simulink model "openloop_on_ramp_mdl"  (Simulink 4.00)
settings: Solver=ode45  StartTime=0.0  StopTime=1097  RelTol=1e-3
values from neighbouring files (symbols this model uses):
  dt = 1    [openloop_on_ramp.m]    (also in same_ord_1_stand_system_new_old_wor.m)
  stm_alpha = 0.0167    [openloop_on_ramp.m]
  stm_ftd = [7 100 120 60   1100 ... (first row only)    [openloop_on_ramp.m]
  stm_ks = 0.031    [openloop_on_ramp.m]
  stm_ks2 = 0.010    (= 0.01)    [openloop_on_ramp.m]
  stm_ks3 = 0.033    [openloop_on_ramp.m]
  stm_ks4 = 0.024    [openloop_on_ramp.m]
  stm_ks5 = 0.025    [openloop_on_ramp.m]
  z0 = 0    [openloop_on_ramp.m]
settings Model: LastModifiedBy=kontorou

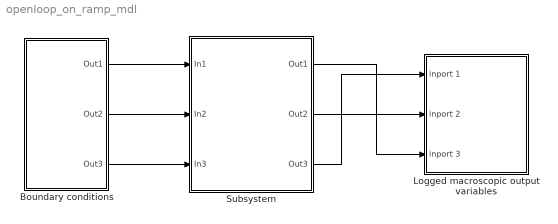
== system openloop_on_ramp_mdl ==
  Boundary conditions : Subsystem
      settings: RTWFcnNameOpts=Auto  RTWFileNameOpts=Auto
      mask Display: disp('Disturbances')
  Logged macroscopic output variables : Subsystem
      settings: RTWFcnNameOpts=Auto  RTWFileNameOpts=Auto
      mask Display: disp('Data')
  Subsystem : Subsystem
      settings: RTWFcnNameOpts=Auto  RTWFileNameOpts=Auto
  wires:
  Subsystem/1(Out1) -> Logged macroscopic output variables/3(inport 3)
  Boundary conditions/1(Out1) -> Subsystem/1(In1)
  Boundary conditions/2(Out2) -> Subsystem/2(In2)
  Subsystem/3(Out3) -> Logged macroscopic output variables/1(inport 1)
  Subsystem/2(Out2) -> Logged macroscopic output variables/2(inport 2)
  Boundary conditions/3(Out3) -> Subsystem/3(In3)

== system openloop_on_ramp_mdl/Boundary conditions ==
  downstream velocity : FromWorkspace  VariableName=[t_in, v_in]  SampleTime=0  OutputAfterFinalValue=Extrapolation
  downstream velocity (km/hour) : ToWorkspace  VariableName=v_in_dt  SampleTime=dt  SaveFormat=Array
  upstream flow : FromWorkspace  VariableName=[t_in, q_in]  SampleTime=0  OutputAfterFinalValue=Extrapolation
  upstream flow1 : FromWorkspace  VariableName=[t_in, q_ramp]  SampleTime=0  OutputAfterFinalValue=Extrapolation
  Out1 : Outport  Port=1
  Out2 : Outport  Port=2
  Out3 : Outport  Port=3
  wires:
  downstream velocity/1 -> Out1/1, downstream velocity (km/hour)/1
  upstream flow/1 -> Out2/1
  upstream flow1/1 -> Out3/1

== system openloop_on_ramp_mdl/Logged macroscopic output variables ==
  inport 1 : Inport  Port=1  LatchInput=off
  inport 2 : Inport  Port=2  LatchInput=off
  inport 3 : Inport  Port=3  LatchInput=off
  Clock : Clock
      settings: DisplayTime=off
  density : ToWorkspace  VariableName=dd  SampleTime=dt  SaveFormat=Array
  flow : ToWorkspace  VariableName=qq  SampleTime=dt  SaveFormat=Array
  time (sample) : ToWorkspace  VariableName=tt  SampleTime=dt  SaveFormat=Array
  velocity : ToWorkspace  VariableName=vv  SampleTime=dt  SaveFormat=Array
  wires:
  inport 3/1 -> velocity/1
  inport 1/1 -> density/1
  inport 2/1 -> flow/1
  Clock/1 -> time (sample)/1

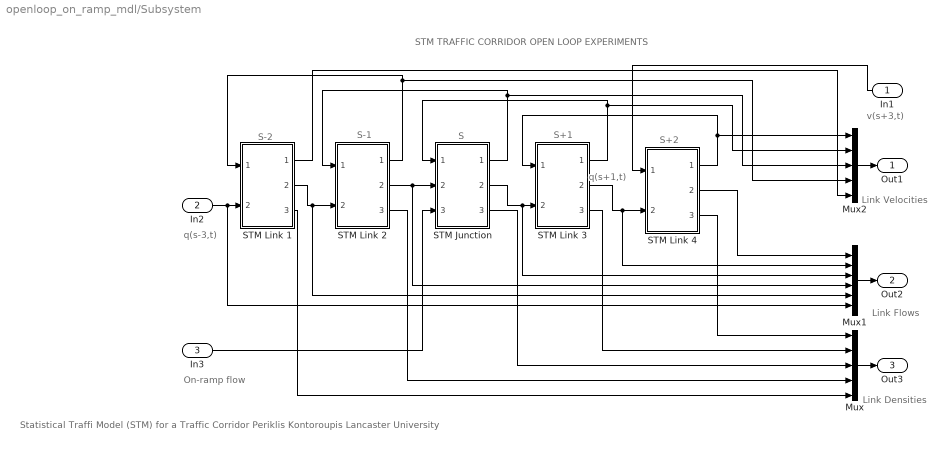
== system openloop_on_ramp_mdl/Subsystem ==
  note: Link
      | Velocities
  note: Link
      | Flows
  note: q(s+1,t)
  note: v(s+3,t)
  note: STM TRAFFIC CORRIDOR OPEN LOOP EXPERIMENTS
  note: On-ramp flow
  note: Link
      | Densities
  note: S-2
  note: S-1
  note: S
  note: S+1
  note: S+2
  note: q(s-3,t)
  note: Statistical Traffi Model (STM)
      | for a Traffic Corridor
      | Periklis Kontoroupis
      | Lancaster University
  In1 : Inport  Orientation=left  Port=1  LatchInput=off
  In2 : Inport  Port=2  LatchInput=off
  In3 : Inport  Port=3  LatchInput=off
  Mux : Mux  Inputs=5
  Mux1 : Mux  Inputs=6
  Mux2 : Mux  Inputs=5
  STM Junction : Subsystem
      settings: RTWFcnNameOpts=Auto  RTWFileNameOpts=Auto
  STM Link 1 : Subsystem
      settings: RTWFcnNameOpts=Auto  RTWFileNameOpts=Auto
  STM Link 2 : Subsystem
      settings: RTWFcnNameOpts=Auto  RTWFileNameOpts=Auto
  STM Link 3 : Subsystem
      settings: RTWFcnNameOpts=Auto  RTWFileNameOpts=Auto
  STM Link 4 : Subsystem
      settings: RTWFcnNameOpts=Auto  RTWFileNameOpts=Auto
  Out1 : Outport  Port=1
  Out2 : Outport  Port=2
  Out3 : Outport  Port=3
  wires:
  STM Link 3/2(link flow (veh/min)) -> STM Link 4/2(upstream flow (veh/min)), Mux1/2
  STM Link 4/1(link velocity (km/hour)) -> STM Link 3/1(downstream velocity (km/hour)), Mux2/1
  Mux1/1 -> Out2/1
  Mux/1 -> Out3/1
  Mux2/1 -> Out1/1
  In2/1 -> STM Link 1/2(upstream flow (veh/min)), Mux1/6
  STM Link 4/2(link flow (veh/min)) -> Mux1/1
  STM Link 4/3(link density (veh/km)) -> Mux/1
  STM Link 3/3(link density (veh/km)) -> Mux/2
  STM Link 1/3(link density (veh/km)) -> Mux/5
  In3/1 -> STM Junction/3(on-ramp flow (veh/min))
  STM Junction/1(link velocity (km/hour)) -> STM Link 2/1(downstream velocity (km/hour)), Mux2/3
  STM Link 2/1(link velocity (km/hour)) -> STM Link 1/1(downstream velocity (km/hour)), Mux2/4
  STM Link 1/2(link flow (veh/min)) -> STM Link 2/2(upstream flow (veh/min)), Mux1/5
  STM Link 2/2(link flow (veh/min)) -> STM Junction/2(upstream flow (veh/min)), Mux1/4
  STM Junction/2(link flow (veh/min)) -> STM Link 3/2(upstream flow (veh/min)), Mux1/3
  STM Link 3/1(link velocity (km/hour)) -> STM Junction/1(downstream velocity (km/hour)), Mux2/2
  STM Link 2/3(link density (veh/km)) -> Mux/4
  STM Junction/3(link density (veh/km)) -> Mux/3
  In1/1 -> STM Link 4/1(downstream velocity (km/hour))
  STM Link 1/1(link velocity (km/hour)) -> Mux2/5

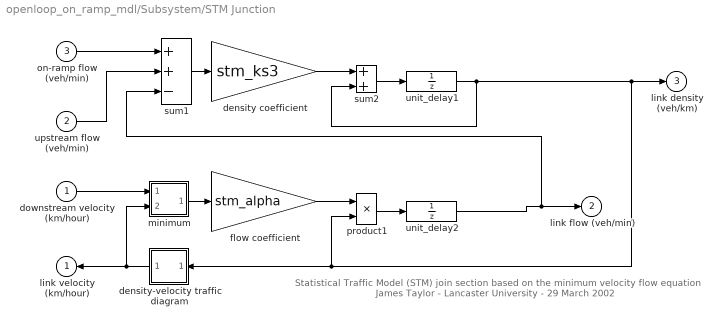
== system openloop_on_ramp_mdl/Subsystem/STM Junction ==
  note: Statistical Traffic Model (STM) join section
      | based on the minimum velocity flow equation
      | James Taylor - Lancaster University - 29 March 2002
  downstream velocity (km/hour) : Inport  Port=1  LatchInput=off
  upstream flow (veh/min) : Inport  Port=2  LatchInput=off
  on-ramp flow (veh/min) : Inport  Port=3  LatchInput=off
  density coefficient : Gain  Gain=stm_ks3  Multiplication=Element-wise(K.*u)  SaturateOnIntegerOverflow=on
  density-velocity traffic diagram : Subsystem  Orientation=left  mask(Fundamental Traffic Diagram){v1=stm_ftd(3,1), v2=stm_ftd(3,2), v3=stm_ftd(3,3), r1=stm_ftd(3,4), r3=stm_ftd(3,5)}
      mask prompts: v1 "Minimum velocity:"; v2 "Critical velocity:"; v3 "Maximum velocity:"; r1 "Critical density:"; r3 "Theoretical density for zero velocity:"
      mask help: Traffic diagram for density-velocity relationship.
      settings: RTWFcnNameOpts=Auto  RTWFileNameOpts=Auto
      mask Help: Connect traffic density to the input and velocity to the output. Based on figure 4 of J. Whittaker, S. Garside and K. Lindveld (1997) Tracking and predicting a network traffic process, International Journal of Forecasting 13, 51-61.
      mask Display: disp('FTD')
  flow coefficient : Gain  Gain=stm_alpha  Multiplication=Element-wise(K.*u)  SaturateOnIntegerOverflow=on
  minimum : Subsystem
      settings: RTWFcnNameOpts=Auto  RTWFileNameOpts=Auto
      mask Type: Minimum
      mask Description: Selects minimum of two inputs.
      mask Help: The output of this block is the minimum of the two input signals.
      mask Display: disp('MIN')
  product1 : Product  Inputs=2  Multiplication=Element-wise(.*)  SaturateOnIntegerOverflow=on
  sum1 : Sum  Inputs=++-  SaturateOnIntegerOverflow=on
  sum2 : Sum  Inputs=++  SaturateOnIntegerOverflow=on
  unit_delay1 : UnitDelay  X0=z0  SampleTime=dt
      settings: RTWStateStorageClass=Auto
  unit_delay2 : UnitDelay  X0=z0  SampleTime=dt
      settings: RTWStateStorageClass=Auto
  link velocity (km/hour) : Outport  Orientation=left  Port=1
  link flow (veh/min) : Outport  Port=2
  link density (veh/km) : Outport  Port=3
  wires:
  on-ramp flow (veh/min)/1 -> sum1/1
  upstream flow (veh/min)/1 -> sum1/2
  flow coefficient/1 -> product1/1
  product1/1 -> unit_delay2/1
  downstream velocity (km/hour)/1 -> minimum/1(inport1)
  unit_delay2/1 -> link flow (veh/min)/1, sum1/3
  sum1/1 -> density coefficient/1
  minimum/1(outport) -> flow coefficient/1
  unit_delay1/1 -> product1/2, density-velocity traffic diagram/1(density), link density (veh/km)/1, sum2/2
  density coefficient/1 -> sum2/1
  sum2/1 -> unit_delay1/1
  density-velocity traffic diagram/1(velocity) -> minimum/2(inport2), link velocity (km/hour)/1

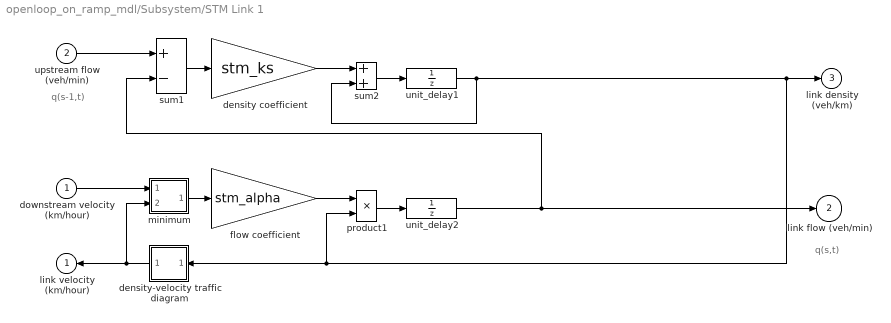
== system openloop_on_ramp_mdl/Subsystem/STM Link 1 ==
  note: q(s-1,t)
  note: q(s,t)
  downstream velocity (km/hour) : Inport  Port=1  LatchInput=off
  upstream flow (veh/min) : Inport  Port=2  LatchInput=off
  density coefficient : Gain  Gain=stm_ks  Multiplication=Element-wise(K.*u)  SaturateOnIntegerOverflow=on
  density-velocity traffic diagram : Subsystem  Orientation=left  mask(Fundamental Traffic Diagram){v1=stm_ftd(1,1), v2=stm_ftd(1,2), v3=stm_ftd(1,3), r1=stm_ftd(1,4), r3=stm_ftd(1,5)}
      mask prompts: v1 "Minimum velocity:"; v2 "Critical velocity:"; v3 "Maximum velocity:"; r1 "Critical density:"; r3 "Theoretical density for zero velocity:"
      mask help: Traffic diagram for density-velocity relationship.
      settings: RTWFcnNameOpts=Auto  RTWFileNameOpts=Auto
      mask Help: Connect traffic density to the input and velocity to the output. Based on figure 4 of J. Whittaker, S. Garside and K. Lindveld (1997) Tracking and predicting a network traffic process, International Journal of Forecasting 13, 51-61.
      mask Display: disp('FTD')
  flow coefficient : Gain  Gain=stm_alpha  Multiplication=Element-wise(K.*u)  SaturateOnIntegerOverflow=on
  minimum : Subsystem
      settings: RTWFcnNameOpts=Auto  RTWFileNameOpts=Auto
      mask Type: Minimum
      mask Description: Selects minimum of two inputs.
      mask Help: The output of this block is the minimum of the two input signals.
      mask Display: disp('MIN')
  product1 : Product  Inputs=2  Multiplication=Element-wise(.*)  SaturateOnIntegerOverflow=on
  sum1 : Sum  Inputs=+-  SaturateOnIntegerOverflow=on
  sum2 : Sum  Inputs=++  SaturateOnIntegerOverflow=on
  unit_delay1 : UnitDelay  X0=z0  SampleTime=dt
      settings: RTWStateStorageClass=Auto
  unit_delay2 : UnitDelay  X0=z0  SampleTime=dt
      settings: RTWStateStorageClass=Auto
  link velocity (km/hour) : Outport  Orientation=left  Port=1
  link flow (veh/min) : Outport  Port=2
  link density (veh/km) : Outport  Port=3
  wires:
  flow coefficient/1 -> product1/1
  product1/1 -> unit_delay2/1
  downstream velocity (km/hour)/1 -> minimum/1(inport1)
  unit_delay2/1 -> sum1/2, link flow (veh/min)/1
  sum1/1 -> density coefficient/1
  minimum/1(outport) -> flow coefficient/1
  unit_delay1/1 -> product1/2, density-velocity traffic diagram/1(density), link density (veh/km)/1, sum2/2
  density coefficient/1 -> sum2/1
  sum2/1 -> unit_delay1/1
  density-velocity traffic diagram/1(velocity) -> minimum/2(inport2), link velocity (km/hour)/1
  upstream flow (veh/min)/1 -> sum1/1

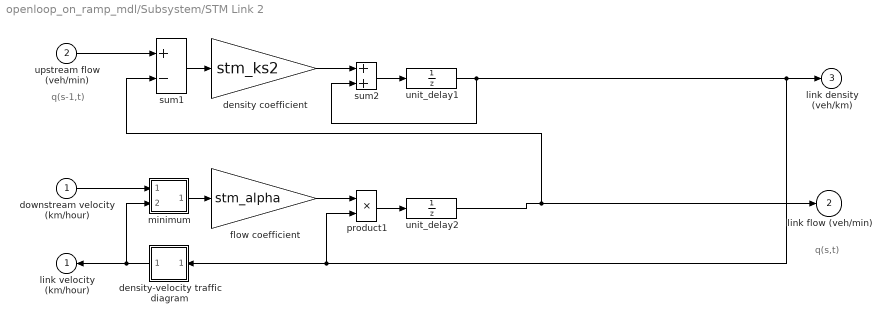
== system openloop_on_ramp_mdl/Subsystem/STM Link 2 ==
  note: q(s-1,t)
  note: q(s,t)
  downstream velocity (km/hour) : Inport  Port=1  LatchInput=off
  upstream flow (veh/min) : Inport  Port=2  LatchInput=off
  density coefficient : Gain  Gain=stm_ks2  Multiplication=Element-wise(K.*u)  SaturateOnIntegerOverflow=on
  density-velocity traffic diagram : Subsystem  Orientation=left  mask(Fundamental Traffic Diagram){v1=stm_ftd(2,1), v2=stm_ftd(2,2), v3=stm_ftd(2,3), r1=stm_ftd(2,4), r3=stm_ftd(2,5)}
      mask prompts: v1 "Minimum velocity:"; v2 "Critical velocity:"; v3 "Maximum velocity:"; r1 "Critical density:"; r3 "Theoretical density for zero velocity:"
      mask help: Traffic diagram for density-velocity relationship.
      settings: RTWFcnNameOpts=Auto  RTWFileNameOpts=Auto
      mask Help: Connect traffic density to the input and velocity to the output. Based on figure 4 of J. Whittaker, S. Garside and K. Lindveld (1997) Tracking and predicting a network traffic process, International Journal of Forecasting 13, 51-61.
      mask Display: disp('FTD')
  flow coefficient : Gain  Gain=stm_alpha  Multiplication=Element-wise(K.*u)  SaturateOnIntegerOverflow=on
  minimum : Subsystem
      settings: RTWFcnNameOpts=Auto  RTWFileNameOpts=Auto
      mask Type: Minimum
      mask Description: Selects minimum of two inputs.
      mask Help: The output of this block is the minimum of the two input signals.
      mask Display: disp('MIN')
  product1 : Product  Inputs=2  Multiplication=Element-wise(.*)  SaturateOnIntegerOverflow=on
  sum1 : Sum  Inputs=+-  SaturateOnIntegerOverflow=on
  sum2 : Sum  Inputs=++  SaturateOnIntegerOverflow=on
  unit_delay1 : UnitDelay  X0=z0  SampleTime=dt
      settings: RTWStateStorageClass=Auto
  unit_delay2 : UnitDelay  X0=z0  SampleTime=dt
      settings: RTWStateStorageClass=Auto
  link velocity (km/hour) : Outport  Orientation=left  Port=1
  link flow (veh/min) : Outport  Port=2
  link density (veh/km) : Outport  Port=3
  wires:
  flow coefficient/1 -> product1/1
  product1/1 -> unit_delay2/1
  downstream velocity (km/hour)/1 -> minimum/1(inport1)
  unit_delay2/1 -> sum1/2, link flow (veh/min)/1
  sum1/1 -> density coefficient/1
  minimum/1(outport) -> flow coefficient/1
  unit_delay1/1 -> product1/2, density-velocity traffic diagram/1(density), link density (veh/km)/1, sum2/2
  density coefficient/1 -> sum2/1
  sum2/1 -> unit_delay1/1
  density-velocity traffic diagram/1(velocity) -> minimum/2(inport2), link velocity (km/hour)/1
  upstream flow (veh/min)/1 -> sum1/1

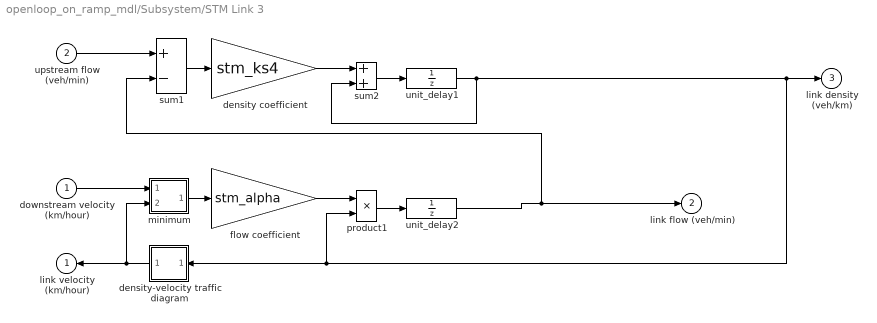
== system openloop_on_ramp_mdl/Subsystem/STM Link 3 ==
  downstream velocity (km/hour) : Inport  Port=1  LatchInput=off
  upstream flow (veh/min) : Inport  Port=2  LatchInput=off
  density coefficient : Gain  Gain=stm_ks4  Multiplication=Element-wise(K.*u)  SaturateOnIntegerOverflow=on
  density-velocity traffic diagram : Subsystem  Orientation=left  mask(Fundamental Traffic Diagram){v1=stm_ftd(4,1), v2=stm_ftd(4,2), v3=stm_ftd(4,3), r1=stm_ftd(4,4), r3=stm_ftd(4,5)}
      mask prompts: v1 "Minimum velocity:"; v2 "Critical velocity:"; v3 "Maximum velocity:"; r1 "Critical density:"; r3 "Theoretical density for zero velocity:"
      mask help: Traffic diagram for density-velocity relationship.
      settings: RTWFcnNameOpts=Auto  RTWFileNameOpts=Auto
      mask Help: Connect traffic density to the input and velocity to the output. Based on figure 4 of J. Whittaker, S. Garside and K. Lindveld (1997) Tracking and predicting a network traffic process, International Journal of Forecasting 13, 51-61.
      mask Display: disp('FTD')
  flow coefficient : Gain  Gain=stm_alpha  Multiplication=Element-wise(K.*u)  SaturateOnIntegerOverflow=on
  minimum : Subsystem
      settings: RTWFcnNameOpts=Auto  RTWFileNameOpts=Auto
      mask Type: Minimum
      mask Description: Selects minimum of two inputs.
      mask Help: The output of this block is the minimum of the two input signals.
      mask Display: disp('MIN')
  product1 : Product  Inputs=2  Multiplication=Element-wise(.*)  SaturateOnIntegerOverflow=on
  sum1 : Sum  Inputs=+-  SaturateOnIntegerOverflow=on
  sum2 : Sum  Inputs=++  SaturateOnIntegerOverflow=on
  unit_delay1 : UnitDelay  X0=z0  SampleTime=dt
      settings: RTWStateStorageClass=Auto
  unit_delay2 : UnitDelay  X0=z0  SampleTime=dt
      settings: RTWStateStorageClass=Auto
  link velocity (km/hour) : Outport  Orientation=left  Port=1
  link flow (veh/min) : Outport  Port=2
  link density (veh/km) : Outport  Port=3
  wires:
  flow coefficient/1 -> product1/1
  product1/1 -> unit_delay2/1
  downstream velocity (km/hour)/1 -> minimum/1(inport1)
  sum1/1 -> density coefficient/1
  minimum/1(outport) -> flow coefficient/1
  unit_delay1/1 -> product1/2, density-velocity traffic diagram/1(density), link density (veh/km)/1, sum2/2
  density coefficient/1 -> sum2/1
  sum2/1 -> unit_delay1/1
  density-velocity traffic diagram/1(velocity) -> minimum/2(inport2), link velocity (km/hour)/1
  unit_delay2/1 -> sum1/2, link flow (veh/min)/1
  upstream flow (veh/min)/1 -> sum1/1

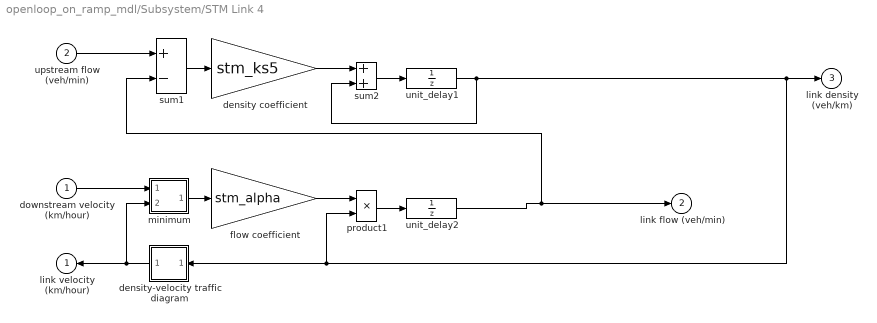
== system openloop_on_ramp_mdl/Subsystem/STM Link 4 ==
  downstream velocity (km/hour) : Inport  Port=1  LatchInput=off
  upstream flow (veh/min) : Inport  Port=2  LatchInput=off
  density coefficient : Gain  Gain=stm_ks5  Multiplication=Element-wise(K.*u)  SaturateOnIntegerOverflow=on
  density-velocity traffic diagram : Subsystem  Orientation=left  mask(Fundamental Traffic Diagram){v1=stm_ftd(5,1), v2=stm_ftd(5,2), v3=stm_ftd(5,3), r1=stm_ftd(5,4), r3=stm_ftd(5,5)}
      mask prompts: v1 "Minimum velocity:"; v2 "Critical velocity:"; v3 "Maximum velocity:"; r1 "Critical density:"; r3 "Theoretical density for zero velocity:"
      mask help: Traffic diagram for density-velocity relationship.
      settings: RTWFcnNameOpts=Auto  RTWFileNameOpts=Auto
      mask Help: Connect traffic density to the input and velocity to the output. Based on figure 4 of J. Whittaker, S. Garside and K. Lindveld (1997) Tracking and predicting a network traffic process, International Journal of Forecasting 13, 51-61.
      mask Display: disp('FTD')
  flow coefficient : Gain  Gain=stm_alpha  Multiplication=Element-wise(K.*u)  SaturateOnIntegerOverflow=on
  minimum : Subsystem
      settings: RTWFcnNameOpts=Auto  RTWFileNameOpts=Auto
      mask Type: Minimum
      mask Description: Selects minimum of two inputs.
      mask Help: The output of this block is the minimum of the two input signals.
      mask Display: disp('MIN')
  product1 : Product  Inputs=2  Multiplication=Element-wise(.*)  SaturateOnIntegerOverflow=on
  sum1 : Sum  Inputs=+-  SaturateOnIntegerOverflow=on
  sum2 : Sum  Inputs=++  SaturateOnIntegerOverflow=on
  unit_delay1 : UnitDelay  X0=z0  SampleTime=dt
      settings: RTWStateStorageClass=Auto
  unit_delay2 : UnitDelay  X0=z0  SampleTime=dt
      settings: RTWStateStorageClass=Auto
  link velocity (km/hour) : Outport  Orientation=left  Port=1
  link flow (veh/min) : Outport  Port=2
  link density (veh/km) : Outport  Port=3
  wires:
  flow coefficient/1 -> product1/1
  product1/1 -> unit_delay2/1
  downstream velocity (km/hour)/1 -> minimum/1(inport1)
  unit_delay2/1 -> sum1/2, link flow (veh/min)/1
  sum1/1 -> density coefficient/1
  minimum/1(outport) -> flow coefficient/1
  unit_delay1/1 -> product1/2, density-velocity traffic diagram/1(density), link density (veh/km)/1, sum2/2
  density coefficient/1 -> sum2/1
  sum2/1 -> unit_delay1/1
  density-velocity traffic diagram/1(velocity) -> minimum/2(inport2), link velocity (km/hour)/1
  upstream flow (veh/min)/1 -> sum1/1

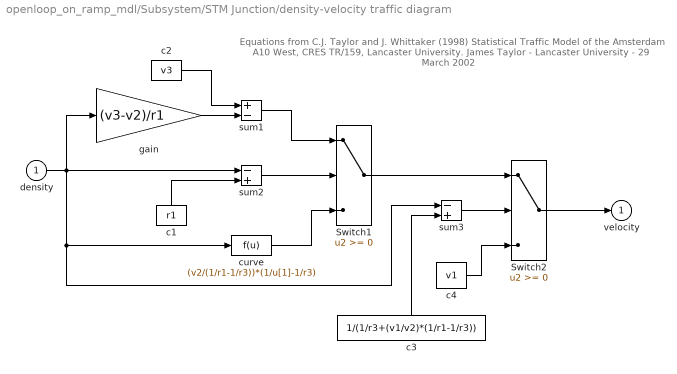
== system openloop_on_ramp_mdl/Subsystem/STM Junction/density-velocity traffic diagram ==
  note: Equations from C.J. Taylor and J. Whittaker (1998) Statistical Traffic Model
      | of the Amsterdam A10 West, CRES TR/159, Lancaster University.
      | James Taylor - Lancaster University - 29 March 2002
  density : Inport  Port=1  LatchInput=off
  Switch1 : Switch  Threshold=0
  Switch2 : Switch  Threshold=0
  c1 : Constant  Orientation=up  Value=r1
  c2 : Constant  Value=v3
  c3 : Constant  Orientation=up  Value=1/(1/r3+(v1/v2)*(1/r1-1/r3))
  c4 : Constant  Value=v1
  curve : Fcn  Expr=(v2/(1/r1-1/r3))*(1/u[1]-1/r3)
  gain : Gain  Gain=(v3-v2)/r1  Multiplication=Element-wise(K.*u)  SaturateOnIntegerOverflow=on
  sum1 : Sum  Inputs=+-  SaturateOnIntegerOverflow=on
  sum2 : Sum  Inputs=-+  SaturateOnIntegerOverflow=on
  sum3 : Sum  Inputs=-+  SaturateOnIntegerOverflow=on
  velocity : Outport  Port=1
  wires:
  c4/1 -> Switch2/3
  sum3/1 -> Switch2/2
  c3/1 -> sum3/2
  curve/1 -> Switch1/3
  Switch1/1 -> Switch2/1
  c1/1 -> sum2/2
  sum2/1 -> Switch1/2
  Switch2/1 -> velocity/1
  c2/1 -> sum1/1
  density/1 -> sum3/1, curve/1, gain/1, sum2/1
  gain/1 -> sum1/2
  sum1/1 -> Switch1/1

== system openloop_on_ramp_mdl/Subsystem/STM Junction/minimum ==
  note: Output is the minimum of the two input signals
      | James Taylor - Lancaster University - 29 March 2002
  inport1 : Inport  Port=1  LatchInput=off
  inport2 : Inport  Port=2  LatchInput=off
  sum1 : Sum  Inputs=-+  SaturateOnIntegerOverflow=on
  switch1 : Switch  Threshold=0
  outport : Outport  Port=1
  wires:
  sum1/1 -> switch1/2
  switch1/1 -> outport/1
  inport2/1 -> switch1/3, sum1/2
  inport1/1 -> switch1/1, sum1/1

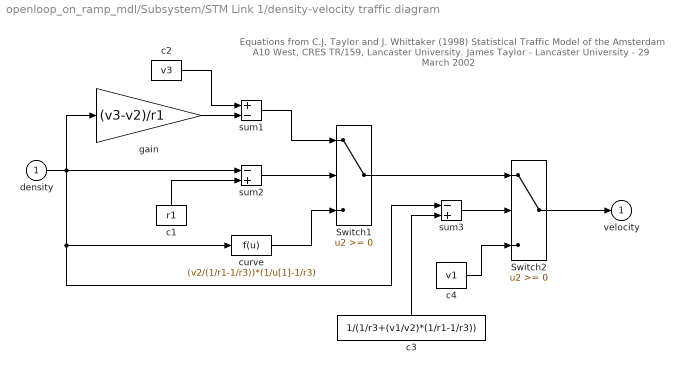
== system openloop_on_ramp_mdl/Subsystem/STM Link 1/density-velocity traffic diagram ==
  note: Equations from C.J. Taylor and J. Whittaker (1998) Statistical Traffic Model
      | of the Amsterdam A10 West, CRES TR/159, Lancaster University.
      | James Taylor - Lancaster University - 29 March 2002
  density : Inport  Port=1  LatchInput=off
  Switch1 : Switch  Threshold=0
  Switch2 : Switch  Threshold=0
  c1 : Constant  Orientation=up  Value=r1
  c2 : Constant  Value=v3
  c3 : Constant  Orientation=up  Value=1/(1/r3+(v1/v2)*(1/r1-1/r3))
  c4 : Constant  Value=v1
  curve : Fcn  Expr=(v2/(1/r1-1/r3))*(1/u[1]-1/r3)
  gain : Gain  Gain=(v3-v2)/r1  Multiplication=Element-wise(K.*u)  SaturateOnIntegerOverflow=on
  sum1 : Sum  Inputs=+-  SaturateOnIntegerOverflow=on
  sum2 : Sum  Inputs=-+  SaturateOnIntegerOverflow=on
  sum3 : Sum  Inputs=-+  SaturateOnIntegerOverflow=on
  velocity : Outport  Port=1
  wires:
  c4/1 -> Switch2/3
  sum3/1 -> Switch2/2
  c3/1 -> sum3/2
  curve/1 -> Switch1/3
  Switch1/1 -> Switch2/1
  c1/1 -> sum2/2
  sum2/1 -> Switch1/2
  Switch2/1 -> velocity/1
  c2/1 -> sum1/1
  density/1 -> sum3/1, curve/1, gain/1, sum2/1
  gain/1 -> sum1/2
  sum1/1 -> Switch1/1

== system openloop_on_ramp_mdl/Subsystem/STM Link 1/minimum ==
  note: Output is the minimum of the two input signals
      | James Taylor - Lancaster University - 29 March 2002
  inport1 : Inport  Port=1  LatchInput=off
  inport2 : Inport  Port=2  LatchInput=off
  sum1 : Sum  Inputs=-+  SaturateOnIntegerOverflow=on
  switch1 : Switch  Threshold=0
  outport : Outport  Port=1
  wires:
  sum1/1 -> switch1/2
  switch1/1 -> outport/1
  inport2/1 -> switch1/3, sum1/2
  inport1/1 -> switch1/1, sum1/1

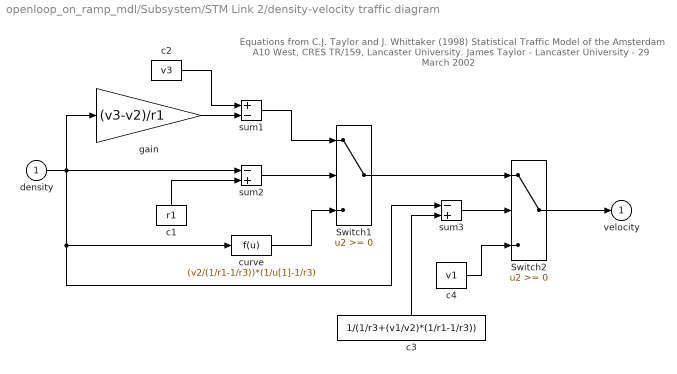
== system openloop_on_ramp_mdl/Subsystem/STM Link 2/density-velocity traffic diagram ==
  note: Equations from C.J. Taylor and J. Whittaker (1998) Statistical Traffic Model
      | of the Amsterdam A10 West, CRES TR/159, Lancaster University.
      | James Taylor - Lancaster University - 29 March 2002
  density : Inport  Port=1  LatchInput=off
  Switch1 : Switch  Threshold=0
  Switch2 : Switch  Threshold=0
  c1 : Constant  Orientation=up  Value=r1
  c2 : Constant  Value=v3
  c3 : Constant  Orientation=up  Value=1/(1/r3+(v1/v2)*(1/r1-1/r3))
  c4 : Constant  Value=v1
  curve : Fcn  Expr=(v2/(1/r1-1/r3))*(1/u[1]-1/r3)
  gain : Gain  Gain=(v3-v2)/r1  Multiplication=Element-wise(K.*u)  SaturateOnIntegerOverflow=on
  sum1 : Sum  Inputs=+-  SaturateOnIntegerOverflow=on
  sum2 : Sum  Inputs=-+  SaturateOnIntegerOverflow=on
  sum3 : Sum  Inputs=-+  SaturateOnIntegerOverflow=on
  velocity : Outport  Port=1
  wires:
  c4/1 -> Switch2/3
  sum3/1 -> Switch2/2
  c3/1 -> sum3/2
  curve/1 -> Switch1/3
  Switch1/1 -> Switch2/1
  c1/1 -> sum2/2
  sum2/1 -> Switch1/2
  Switch2/1 -> velocity/1
  c2/1 -> sum1/1
  density/1 -> sum3/1, curve/1, gain/1, sum2/1
  gain/1 -> sum1/2
  sum1/1 -> Switch1/1

== system openloop_on_ramp_mdl/Subsystem/STM Link 2/minimum ==
  note: Output is the minimum of the two input signals
      | James Taylor - Lancaster University - 29 March 2002
  inport1 : Inport  Port=1  LatchInput=off
  inport2 : Inport  Port=2  LatchInput=off
  sum1 : Sum  Inputs=-+  SaturateOnIntegerOverflow=on
  switch1 : Switch  Threshold=0
  outport : Outport  Port=1
  wires:
  sum1/1 -> switch1/2
  switch1/1 -> outport/1
  inport2/1 -> switch1/3, sum1/2
  inport1/1 -> switch1/1, sum1/1

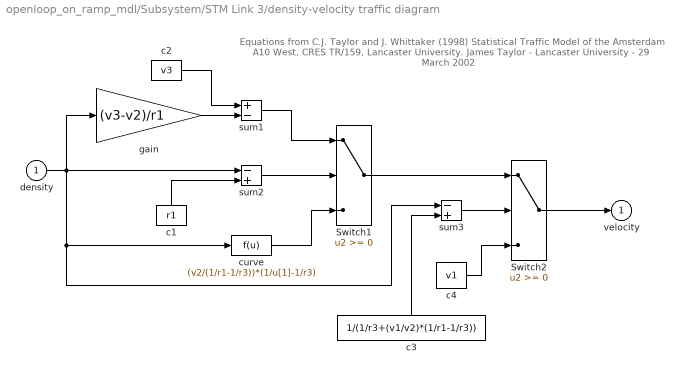
== system openloop_on_ramp_mdl/Subsystem/STM Link 3/density-velocity traffic diagram ==
  note: Equations from C.J. Taylor and J. Whittaker (1998) Statistical Traffic Model
      | of the Amsterdam A10 West, CRES TR/159, Lancaster University.
      | James Taylor - Lancaster University - 29 March 2002
  density : Inport  Port=1  LatchInput=off
  Switch1 : Switch  Threshold=0
  Switch2 : Switch  Threshold=0
  c1 : Constant  Orientation=up  Value=r1
  c2 : Constant  Value=v3
  c3 : Constant  Orientation=up  Value=1/(1/r3+(v1/v2)*(1/r1-1/r3))
  c4 : Constant  Value=v1
  curve : Fcn  Expr=(v2/(1/r1-1/r3))*(1/u[1]-1/r3)
  gain : Gain  Gain=(v3-v2)/r1  Multiplication=Element-wise(K.*u)  SaturateOnIntegerOverflow=on
  sum1 : Sum  Inputs=+-  SaturateOnIntegerOverflow=on
  sum2 : Sum  Inputs=-+  SaturateOnIntegerOverflow=on
  sum3 : Sum  Inputs=-+  SaturateOnIntegerOverflow=on
  velocity : Outport  Port=1
  wires:
  c4/1 -> Switch2/3
  sum3/1 -> Switch2/2
  c3/1 -> sum3/2
  curve/1 -> Switch1/3
  Switch1/1 -> Switch2/1
  c1/1 -> sum2/2
  sum2/1 -> Switch1/2
  Switch2/1 -> velocity/1
  c2/1 -> sum1/1
  density/1 -> sum3/1, curve/1, gain/1, sum2/1
  gain/1 -> sum1/2
  sum1/1 -> Switch1/1

== system openloop_on_ramp_mdl/Subsystem/STM Link 3/minimum ==
  note: Output is the minimum of the two input signals
      | James Taylor - Lancaster University - 29 March 2002
  inport1 : Inport  Port=1  LatchInput=off
  inport2 : Inport  Port=2  LatchInput=off
  sum1 : Sum  Inputs=-+  SaturateOnIntegerOverflow=on
  switch1 : Switch  Threshold=0
  outport : Outport  Port=1
  wires:
  sum1/1 -> switch1/2
  switch1/1 -> outport/1
  inport2/1 -> switch1/3, sum1/2
  inport1/1 -> switch1/1, sum1/1

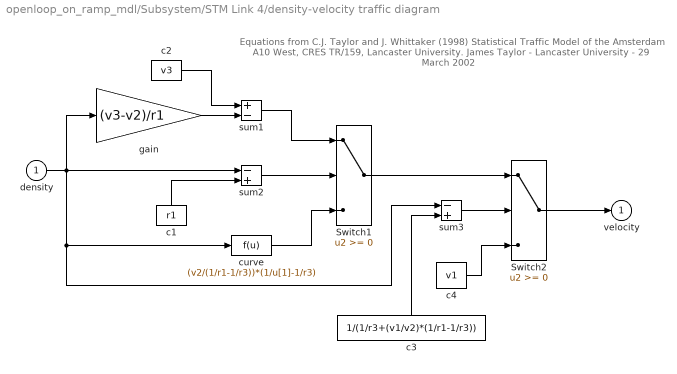
== system openloop_on_ramp_mdl/Subsystem/STM Link 4/density-velocity traffic diagram ==
  note: Equations from C.J. Taylor and J. Whittaker (1998) Statistical Traffic Model
      | of the Amsterdam A10 West, CRES TR/159, Lancaster University.
      | James Taylor - Lancaster University - 29 March 2002
  density : Inport  Port=1  LatchInput=off
  Switch1 : Switch  Threshold=0
  Switch2 : Switch  Threshold=0
  c1 : Constant  Orientation=up  Value=r1
  c2 : Constant  Value=v3
  c3 : Constant  Orientation=up  Value=1/(1/r3+(v1/v2)*(1/r1-1/r3))
  c4 : Constant  Value=v1
  curve : Fcn  Expr=(v2/(1/r1-1/r3))*(1/u[1]-1/r3)
  gain : Gain  Gain=(v3-v2)/r1  Multiplication=Element-wise(K.*u)  SaturateOnIntegerOverflow=on
  sum1 : Sum  Inputs=+-  SaturateOnIntegerOverflow=on
  sum2 : Sum  Inputs=-+  SaturateOnIntegerOverflow=on
  sum3 : Sum  Inputs=-+  SaturateOnIntegerOverflow=on
  velocity : Outport  Port=1
  wires:
  c4/1 -> Switch2/3
  sum3/1 -> Switch2/2
  c3/1 -> sum3/2
  curve/1 -> Switch1/3
  Switch1/1 -> Switch2/1
  c1/1 -> sum2/2
  sum2/1 -> Switch1/2
  Switch2/1 -> velocity/1
  c2/1 -> sum1/1
  density/1 -> sum3/1, curve/1, gain/1, sum2/1
  gain/1 -> sum1/2
  sum1/1 -> Switch1/1

== system openloop_on_ramp_mdl/Subsystem/STM Link 4/minimum ==
  note: Output is the minimum of the two input signals
      | James Taylor - Lancaster University - 29 March 2002
  inport1 : Inport  Port=1  LatchInput=off
  inport2 : Inport  Port=2  LatchInput=off
  sum1 : Sum  Inputs=-+  SaturateOnIntegerOverflow=on
  switch1 : Switch  Threshold=0
  outport : Outport  Port=1
  wires:
  sum1/1 -> switch1/2
  switch1/1 -> outport/1
  inport2/1 -> switch1/3, sum1/2
  inport1/1 -> switch1/1, sum1/1
